simulink subsystem "boundary_cell_givens"  (R2020b)
settings: Solver=VariableStepAuto  StartTime=0.0  StopTime=10.0  RelTol=1e-3
values from neighbouring files (symbols this model uses):
  lambda = 0.995    [env_sim_setup.m]
  sigma = 1e-6    (= 1e-06)    [env_sim_setup.m]
undefined symbols (not defined in the file or in its folder): magnitude
libraries: simulink x1, hdlsllib x1
settings Model: Creator=johngentile  LastModifiedBy=jgentile

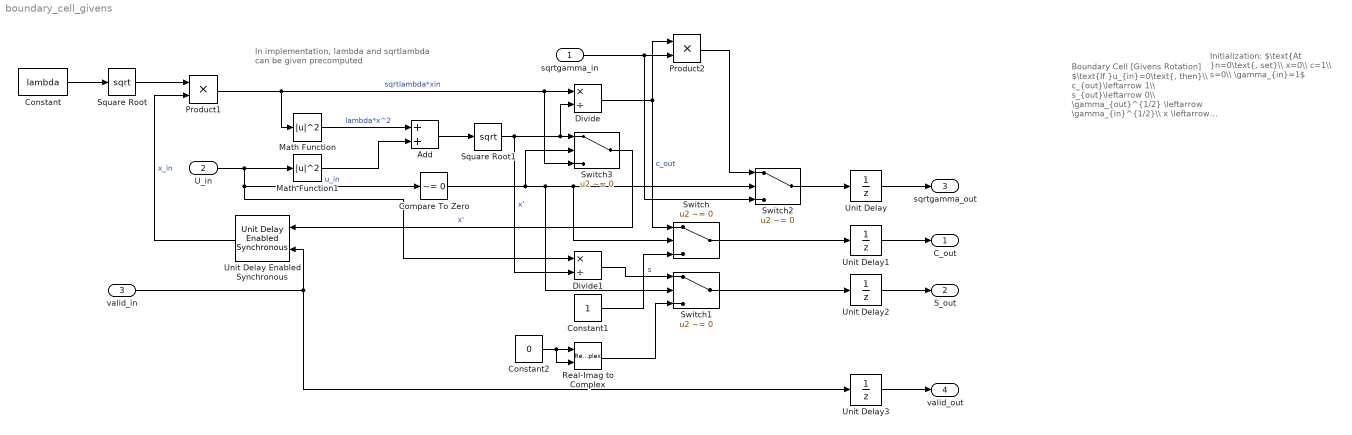
== system boundary_cell_givens ==
  note: In implementation, lambda and sqrtlambda
      | can be given precomputed
  note: Initialization:
      | $\text{At }n=0\text{, set}\\ x=0\\ c=1\\ s=0\\ \gamma_{in}=1$
  note: Boundary Cell [Givens Rotation]
      | $\text{If }u_{in}=0\text{, then}\\ c_{out}\leftarrow 1\\ s_{out}\leftarrow 0\\ \gamma_{out}^{1/2} \leftarrow \gamma_{in}^{1/2}\\ x \leftarrow \lambda^{1/2}x\\ \text{Otherwise,}\\ x'\leftarrow\sqrt{\lambda x^{2} + |u_{in}|^{2}}\\ c_{out}\leftarrow \frac{\lambda^{1/2}x}{x'}\\ s_{out}\leftarrow \frac{u_{in}}{x'}\\ x\leftarrow x'\\ \gamma_{out}^{1/2} \leftarrow c\gamma_{in}^{1/2}\\$
  sqrtgamma_in : Inport
  U_in : Inport  Port=2
      settings: SignalType=complex
  valid_in : Inport  Port=3
  Add : Sum
  Compare To Zero : simulink/Logic and Bit Operations/Compare To Zero  relop=~=  OutDataTypeStr=boolean
  Constant : Constant  Value=lambda
  Constant1 : Constant
  Constant2 : Constant  Value=0
  Divide : Product  Inputs=*/
  Divide1 : Product  Inputs=*/
  Math Function : Math  Operator=magnitude^2  SaturateOnIntegerOverflow=on
  Math Function1 : Math  Operator=magnitude^2  SaturateOnIntegerOverflow=on
  Product1 : Product
  Product2 : Product
  Real-Imag to Complex : RealImagToComplex
  Square Root : Sqrt  SaturateOnIntegerOverflow=on
  Square Root1 : Sqrt  SaturateOnIntegerOverflow=on
  Switch{,1..3} (4 alike) : Switch  Criteria=u2 ~= 0
  Unit Delay{,1..3} (4 alike) : UnitDelay  SampleTime=-1  HasFrameUpgradeWarning=on
  Unit Delay Enabled Synchronous : hdlsllib/Discrete/Unit Delay Enabled Synchronous  InitialCondition=sigma  SampleTime=-1
      settings: SourceProductBaseCode=SL
  C_out : Outport
  S_out : Outport  Port=2
      settings: SignalType=complex
  sqrtgamma_out : Outport  Port=3
  valid_out : Outport  Port=4
  wires:
  U_in/1 -> Compare To Zero/1, Divide1/1, Math Function1/1  "u_in"
  Square Root1/1 -> Divide1/2, Switch3/1, Divide/2  "x'"
  sqrtgamma_in/1 -> Product2/2, Switch2/3
  Product1/1 -> Divide/1, Switch3/3, Math Function/1  "sqrtlambda*xin"
  Unit Delay Enabled Synchronous/1 -> Product1/2  "x_in"
  Constant2/1 -> Real-Imag to Complex/1, Real-Imag to Complex/2
  Compare To Zero/1 -> Switch3/2, Switch1/2, Switch2/2, Switch/2
  Constant1/1 -> Switch/3
  Product2/1 -> Switch2/1
  Divide/1 -> Product2/1, Switch/1  "c_out"
  Add/1 -> Square Root1/1
  Switch3/1 -> Unit Delay Enabled Synchronous/1  "x'"
  Math Function1/1 -> Add/2
  Real-Imag to Complex/1 -> Switch1/3
  Divide1/1 -> Switch1/1  "s"
  Math Function/1 -> Add/1  "lambda*x^2"
  Constant/1 -> Square Root/1
  Square Root/1 -> Product1/1
  Switch2/1 -> Unit Delay/1
  Unit Delay/1 -> sqrtgamma_out/1
  Switch/1 -> Unit Delay1/1
  Unit Delay1/1 -> C_out/1
  Switch1/1 -> Unit Delay2/1
  Unit Delay2/1 -> S_out/1
  valid_in/1 -> Unit Delay3/1, Unit Delay Enabled Synchronous/2
  Unit Delay3/1 -> valid_out/1
